simulink model "model"  (R2023a)
settings: Solver=VariableStepAuto  StartTime=0.0  StopTime=10.0  RelTol=1e-3
undefined symbols (not defined in the file): map
libraries: slpidlib x2, robotmobilelib x1
settings Model: SimulationMode=rapid-accelerator  Creator=Pawel  LastModifiedBy=Pawel
settings SolverCC: AllowMultiTaskInputOutput=on  ConcurrentTasks=on

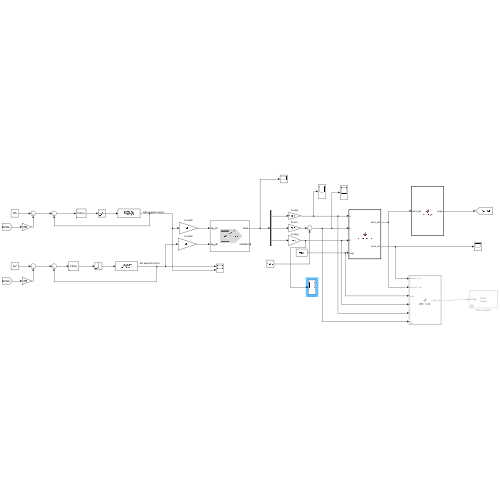
[thumbnail: Simulink's stored preview of the top-level diagram]
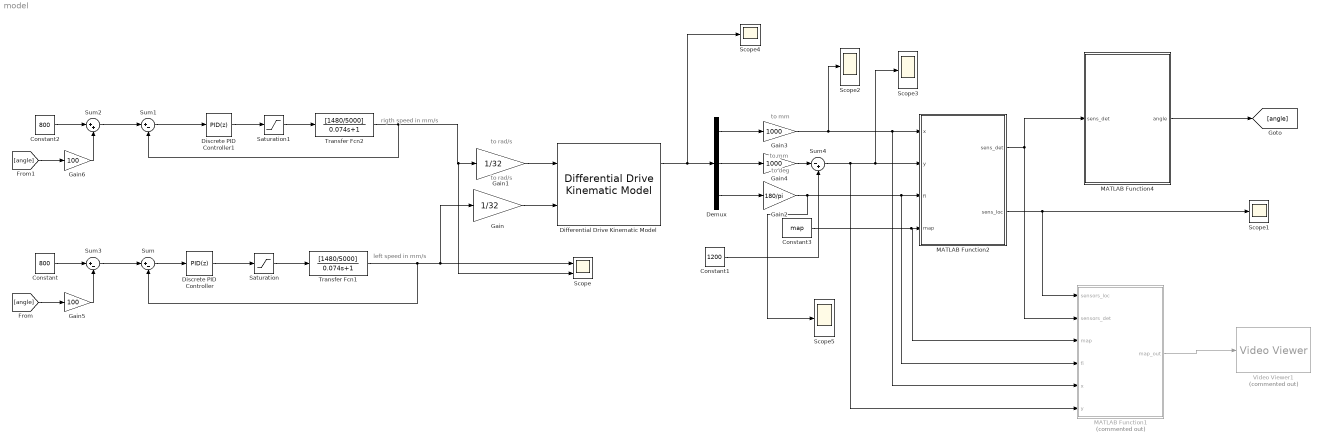
== system model ==
  note: to mm
  note: to rad/s
  note: left speed in mm/s
  note: rigth speed in mm/s
  note: to rad/s
  note: to mm
  note: to deg
  Constant : Constant  Value=800
  Constant1 : Constant  Value=1200
  Constant2 : Constant  Value=800
  Constant3 : Constant  Value=map
  Demux : Demux  Outputs=3
  Differential Drive Kinematic Model : robotmobilelib/Differential Drive Kinematic Model  VehicleInputs=Wheel Speeds  WheelRadius=0.032  WheelSpeedRange=[-inf inf]  TrackWidth=0.12  InitialState=[500/1000; 700/1000; -pi/2]  SimulateUsing=Interpreted execution
  Discrete PID Controller : slpidlib/PID Controller  Controller=PID  Form=Parallel  TimeDomain=Discrete-time  UseExternalTs=off  SampleTime=0.0005  IntegratorMethod=Backward Euler  FilterMethod=Forward Euler  ControllerParametersSource=internal  P=8  I=0.05  UseKiTs=on  D=0  N=100  UseFilter=off  TunerSelectOption=Transfer Function Based (PID Tuner App)  InitialConditionSource=internal  InitialConditionForIntegrator=0  InitialConditionForFilter=0  DifferentiatorICPrevScaledInput=0  ExternalReset=none  TrackingMode=off  Kt=1  LimitOutput=off  SatLimitsSource=internal  UpperSaturationLimit=inf  LowerSaturationLimit=-inf  LinearizeAsGain=off  AntiWindupMode=none  Kb=1  LimitIntegrator=off  UpperIntegratorSaturationLimit=inf  LowerIntegratorSaturationLimit=-inf  POutMin=[]  POutMax=[]  IOutMin=[]  IOutMax=[]  DOutMin=[]  DOutMax=[]  NOutMin=[]  NOutMax=[]  SumOutMin=[]  SumOutMax=[]  SaturationOutMin=[]  SaturationOutMax=[]  PParamMin=[]  PParamMax=[]  IParamMin=[]  IParamMax=[]  DParamMin=[]  DParamMax=[]  NParamMin=[]  NParamMax=[]  KbParamMin=[]  KbParamMax=[]  KtParamMin=[]  KtParamMax=[]  KbOutMin=[]  KbOutMax=[]  KtOutMin=[]  KtOutMax=[]  IntegratorOutMin=[]  IntegratorOutMax=[]  FilterOutMin=[]  FilterOutMax=[]  SumI1OutMin=[]  SumI1OutMax=[]  SumI2OutMin=[]  SumI2OutMax=[]  SumI3OutMin=[]  SumI3OutMax=[]  SumI4OutMin=[]  SumI4OutMax=[]  SumDOutMin=[]  SumDOutMax=[]  DifferentiatorOutMin=[]  DifferentiatorOutMax=[]  FilterDiffOutCoefMin=[]  FilterDiffOutCoefMax=[]  ReciprocalOutMin=[]  ReciprocalOutMax=[]  SumDenOutMin=[]  SumDenOutMax=[]  SumNumOutMin=[]  SumNumOutMax=[]  DivideOutMin=[]  DivideOutMax=[]  UdiffTsProdOutMin=[]  UdiffTsProdOutMax=[]  NTsProdOutMin=[]  NTsProdOutMax=[]  UintegralTsProdOutMin=[]  UintegralTsProdOutMax=[]  UngainTsProdOutMin=[]  UngainTsProdOutMax=[]  ClampingZeroOutDataTypeStr=Inherit: Inherit via back propagation  ClampingZeroOutMin=[]  ClampingZeroOutMax=[]  FilterDenConstantOutDataTypeStr=Inherit: Inherit via back propagation  FilterDenConstantOutMin=[]  FilterDenConstantOutMax=[]  PCopyOutDataTypeStr=Inherit: Inherit via back propagation  PCopyOutMin=[]  PCopyOutMax=[]  NCopyOutDataTypeStr=Inherit: Inherit via back propagation  NCopyOutMin=[]  NCopyOutMax=[]  IntegratorContinuousStateAttributes=''  IntegratorStateMustResolveToSignalObject=off  IntegratorRTWStateStorageClass=Auto  FilterContinuousStateAttributes=''  FilterStateMustResolveToSignalObject=off  FilterRTWStateStorageClass=Auto  ParallelPVariant=InternalParameters  IdealPVariant=Disabled  IVariant=InternalParameters  DVariant=InternalParameters  IntegratorVariant=Discrete  SatVariant=Disabled  AWVariant=Passthrough  PCopyVariant=Disabled  TRVariant=Disabled  FdbkBlocksVariant=Forward  IdealPFdbkVariant=Disabled  SatFdbkVariant=Disabled  DerivativeFilterVariant=Differentiator  NVariant=Passthrough  NCopyVariant=Disabled_SignalSpec  FilterICVariant=InternalICsDifferentiator  IntegratorICVariant=InternalICs  ExternalResetVariant=Disabled  TRSumVariant=Passthrough  SumFdbkVariant=Disabled  SumVariant=Sum_PID  TsampFilterVariant=InternalTs  TsampNgainVariant=Passthrough  TsampIntegralVariant=Disabled_SignalSpec  ExternalSaturationOutDataTypeStr=Inherit: Same as second input
      settings: LibrarySourceBlock=simulink/Discrete/Discrete PID Controller
  Discrete PID Controller1 : slpidlib/PID Controller  Controller=PID  Form=Parallel  TimeDomain=Discrete-time  UseExternalTs=off  SampleTime=0.0005  IntegratorMethod=Backward Euler  FilterMethod=Forward Euler  ControllerParametersSource=internal  P=8  I=0.05  UseKiTs=on  D=0  N=100  UseFilter=off  TunerSelectOption=Transfer Function Based (PID Tuner App)  InitialConditionSource=internal  InitialConditionForIntegrator=0  InitialConditionForFilter=0  DifferentiatorICPrevScaledInput=0  ExternalReset=none  TrackingMode=off  Kt=1  LimitOutput=off  SatLimitsSource=internal  UpperSaturationLimit=inf  LowerSaturationLimit=-inf  LinearizeAsGain=off  AntiWindupMode=none  Kb=1  LimitIntegrator=off  UpperIntegratorSaturationLimit=inf  LowerIntegratorSaturationLimit=-inf  POutMin=[]  POutMax=[]  IOutMin=[]  IOutMax=[]  DOutMin=[]  DOutMax=[]  NOutMin=[]  NOutMax=[]  SumOutMin=[]  SumOutMax=[]  SaturationOutMin=[]  SaturationOutMax=[]  PParamMin=[]  PParamMax=[]  IParamMin=[]  IParamMax=[]  DParamMin=[]  DParamMax=[]  NParamMin=[]  NParamMax=[]  KbParamMin=[]  KbParamMax=[]  KtParamMin=[]  KtParamMax=[]  KbOutMin=[]  KbOutMax=[]  KtOutMin=[]  KtOutMax=[]  IntegratorOutMin=[]  IntegratorOutMax=[]  FilterOutMin=[]  FilterOutMax=[]  SumI1OutMin=[]  SumI1OutMax=[]  SumI2OutMin=[]  SumI2OutMax=[]  SumI3OutMin=[]  SumI3OutMax=[]  SumI4OutMin=[]  SumI4OutMax=[]  SumDOutMin=[]  SumDOutMax=[]  DifferentiatorOutMin=[]  DifferentiatorOutMax=[]  FilterDiffOutCoefMin=[]  FilterDiffOutCoefMax=[]  ReciprocalOutMin=[]  ReciprocalOutMax=[]  SumDenOutMin=[]  SumDenOutMax=[]  SumNumOutMin=[]  SumNumOutMax=[]  DivideOutMin=[]  DivideOutMax=[]  UdiffTsProdOutMin=[]  UdiffTsProdOutMax=[]  NTsProdOutMin=[]  NTsProdOutMax=[]  UintegralTsProdOutMin=[]  UintegralTsProdOutMax=[]  UngainTsProdOutMin=[]  UngainTsProdOutMax=[]  ClampingZeroOutDataTypeStr=Inherit: Inherit via back propagation  ClampingZeroOutMin=[]  ClampingZeroOutMax=[]  FilterDenConstantOutDataTypeStr=Inherit: Inherit via back propagation  FilterDenConstantOutMin=[]  FilterDenConstantOutMax=[]  PCopyOutDataTypeStr=Inherit: Inherit via back propagation  PCopyOutMin=[]  PCopyOutMax=[]  NCopyOutDataTypeStr=Inherit: Inherit via back propagation  NCopyOutMin=[]  NCopyOutMax=[]  IntegratorContinuousStateAttributes=''  IntegratorStateMustResolveToSignalObject=off  IntegratorRTWStateStorageClass=Auto  FilterContinuousStateAttributes=''  FilterStateMustResolveToSignalObject=off  FilterRTWStateStorageClass=Auto  ParallelPVariant=InternalParameters  IdealPVariant=Disabled  IVariant=InternalParameters  DVariant=InternalParameters  IntegratorVariant=Discrete  SatVariant=Disabled  AWVariant=Passthrough  PCopyVariant=Disabled  TRVariant=Disabled  FdbkBlocksVariant=Forward  IdealPFdbkVariant=Disabled  SatFdbkVariant=Disabled  DerivativeFilterVariant=Differentiator  NVariant=Passthrough  NCopyVariant=Disabled_SignalSpec  FilterICVariant=InternalICsDifferentiator  IntegratorICVariant=InternalICs  ExternalResetVariant=Disabled  TRSumVariant=Passthrough  SumFdbkVariant=Disabled  SumVariant=Sum_PID  TsampFilterVariant=InternalTs  TsampNgainVariant=Passthrough  TsampIntegralVariant=Disabled_SignalSpec  ExternalSaturationOutDataTypeStr=Inherit: Same as second input
      settings: LibrarySourceBlock=simulink/Discrete/Discrete PID Controller
  Gain : Gain  Gain=1/32
  Gain1 : Gain  Gain=1/32
  Gain2 : Gain  Gain=180/pi
  Gain3 : Gain  Gain=1000
  Gain4 : Gain  Gain=1000
  Gain5 : Gain  Gain=100
  Gain6 : Gain  Gain=100
  MATLAB Function1 : MATLAB Function  Commented=on  TreatAsAtomicUnit=on
  MATLAB Function2 : MATLAB Function  TreatAsAtomicUnit=on
  MATLAB Function4 : MATLAB Function  TreatAsAtomicUnit=on
  Saturation : Saturate  UpperLimit=10000  LowerLimit=-10000
  Saturation1 : Saturate  UpperLimit=10000  LowerLimit=-10000
  Scope : Scope  NumInputPorts=2
  Scope{1..5} (5 alike) : Scope
  Sum : Sum  Inputs=|+-
  Sum1 : Sum  Inputs=|+-
  Sum2 : Sum  Inputs=|++
  Sum3 : Sum  Inputs=|+-
  Sum4 : Sum  Inputs=|-+
  Transfer Fcn1 : TransferFcn  Numerator=[1480/5000]  Denominator=[0.074 1]
  Transfer Fcn2 : TransferFcn  Numerator=[1480/5000]  Denominator=[0.074 1]
  Video Viewer1 : VideoViewer  Commented=on  FigPos=[-19 1039 1920 856]
  wires:
  Transfer Fcn1/1 -> Gain/1, Scope/1, Sum/2
  Sum/1 -> Discrete PID Controller/1
  Sum1/1 -> Discrete PID Controller1/1
  Transfer Fcn2/1 -> Sum1/2, Scope/2, Gain1/1
  Demux/1 -> Gain3/1
  Demux/2 -> Gain4/1
  Discrete PID Controller1/1 -> Saturation1/1
  Discrete PID Controller/1 -> Saturation/1
  Saturation/1 -> Transfer Fcn1/1
  Saturation1/1 -> Transfer Fcn2/1
  Gain/1 -> Differential Drive Kinematic Model/2
  Gain1/1 -> Differential Drive Kinematic Model/1
  Differential Drive Kinematic Model/1 -> Scope4/1, Demux/1
  Demux/3 -> Gain2/1
  Gain2/1 -> Scope5/1, MATLAB Function2/3(fi), MATLAB Function1/4(fi)
  Gain3/1 -> Scope2/1, MATLAB Function1/5(x), MATLAB Function2/1(x)
  Constant3/1 -> MATLAB Function1/3(map), MATLAB Function2/4(map)
  MATLAB Function2/2(sens_loc) -> MATLAB Function1/1(sensors_loc), Scope1/1
  MATLAB Function1/1(map_out) -> Video Viewer1/1
  MATLAB Function2/1(sens_det) -> MATLAB Function1/2(sensors_det), MATLAB Function4/1(sens_det)
  Constant2/1 -> Sum2/1
  Sum2/1 -> Sum1/1
  Constant/1 -> Sum3/1
  Sum3/1 -> Sum/1
  MATLAB Function4/1(angle) -> [angle]
  [angle] -> Gain5/1
  [angle] -> Gain6/1
  Gain5/1 -> Sum3/2
  Gain6/1 -> Sum2/2
  Sum4/1 -> MATLAB Function1/6(y), Scope3/1, MATLAB Function2/2(y)
  Gain4/1 -> Sum4/1
  Constant1/1 -> Sum4/2

== matlab function model/MATLAB Function1 ==
  data: sensors_loc input; map_out output; sensors_det input; map input; fi input; x input; y input
function map_out  = draw_robot(sensors_loc, sensors_det, map, fi,x ,y)

map_out = uint8(map)*255;


rM = [cosd(fi), -sind(fi);
      sind(fi),  cosd(fi)];

wheel_left_v = [0, 50] * rM;
wheel_right_v = [0, -50] * rM;


sensors_loc = int32(sensors_loc);
for i = 1:10
    if(sensors_det(i) == 1)
        for j = -7:7
            for k = -7:7
                if ((j*j + k*k) < 36)
                    s_x = sensors_loc(i, 1)+j;
                    s_y = sensors_loc(i, 2)+k;
                    map_out(s_x, s_y) = 200;
                end
            end
        end
    else
        for j = -7:7
            for k = -7:7
                if ((j*j + k*k) < 36)
                    s_x = sensors_loc(i, 1)+j;
                    s_y = sensors_loc(i, 2)+k;
                    map_out(s_x, s_y) = 50;
                end
            end
        end
    end
end


map_out(int32(x)-5:int32(x)+5, int32(y)-5:int32(y)+5) = 100;
wh_loc_lx = wheel_left_v(1) + int32(x);
wh_loc_ly = wheel_left_v(2) + int32(y);
wh_loc_rx = wheel_right_v(1) + int32(x);
wh_loc_ry = wheel_right_v(2) + int32(y);
map_out(wh_loc_lx-2:wh_loc_lx+2, wh_loc_ly-2:wh_loc_ly+2) = 100;
map_out(wh_loc_rx-2:wh_loc_rx+2, wh_loc_ry-2:wh_loc_ry+2) = 100;

== matlab function model/MATLAB Function4 ==
  data: angle output; sens_det input
function angle  = est_angle(sens_det)
angle = 0;
for i=1:10
    if(sens_det(i) == 1)
        if(i <= 5)
            angle = 5*(i-6);
        else
            angle = 5*(i-5);
        end
    end
end

== matlab function model/MATLAB Function2 ==
  data: x input; sens_det output; y input; fi input; map input; sens_loc output
function [sens_det, sens_loc] = sensor_detec(x, y, fi, map)
sensor_loc = [145 -71;
              147, -59;
              150, -41;
              154, -25;
              157, -12;
              157, 12;
              154, 25;
              150, 41;
              147, 59;
              145, 71];
rM = [cosd(fi), -sind(fi);
      sind(fi),  cosd(fi)];

sens_det = zeros(10);
sens_rot = zeros([10,2]);
on_map_loc = zeros([10,2]);

for i = 1:10
    sens_rot(i,:) = sensor_loc(i,:) * rM;
    on_map_loc(i,:) = [sens_rot(i,1) + x, sens_rot(i,2) + y];
    if(map(uint32(on_map_loc(i,1)), uint32(on_map_loc(i,2))) == 0)
        sens_det(i) = 1;
    end
end

sens_loc = int32(on_map_loc);
